simulink model "LV"  (R2016a)
settings: Solver=VariableStepAuto  StartTime=0.0  StopTime=10.0  RelTol=1e-3
libraries: powerlib x22
settings Model: Creator=Hp  LastModifiedBy=Hp

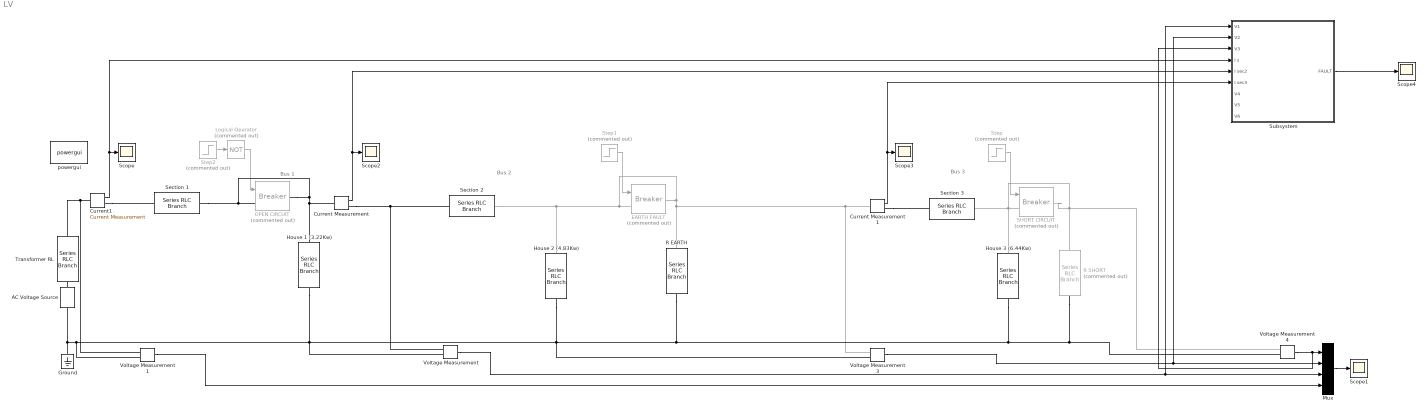
== system LV ==
  note: Bus 3
  note: Bus 2
  note: Bus 1
  AC Voltage Source : powerlib/Electrical Sources/AC Voltage Source  Amplitude=230  Phase=0  Frequency=50  SampleTime=0  Measurements=Voltage  BusType=swing  Pref=10e3  Qref=0  Qmin=-inf  Qmax=+inf
  Current Measurement : powerlib/Measurements/Current Measurement  PhasorSimulation=off  OutputType=Complex  PSBequivalent=0
  Current Measurement1 : powerlib/Measurements/Current Measurement  PhasorSimulation=off  OutputType=Complex  PSBequivalent=0
  Current1 : powerlib/Measurements/Current Measurement  PhasorSimulation=off  OutputType=Complex  PSBequivalent=0
  EARTH FAULT : powerlib/Elements/Breaker  Commented=on  InitialState=0  SwitchingTimes="[1/60  5/60]"  External=on  BreakerResistance=0.05  SnubberResistance=1e6  SnubberCapacitance=inf  Measurements=None  MoreParameters=on  NoBreakLoop=off
  Ground : powerlib/Elements/Ground  LConnTagsString=a
  House 1 (3.22Kw) : powerlib/Elements/Series RLC Branch  LConnTagsString=__new0  RConnTagsString=__new0  BranchType=RL  Resistance=16.43  Inductance=0.02497  SetiL0=off  InitialCurrent=0  Capacitance=1e-6  Setx0=off  InitialVoltage=0  Measurements=None
  House 2 (4.83Kw) : powerlib/Elements/Series RLC Branch  LConnTagsString=__new0  RConnTagsString=__new0  BranchType=RL  Resistance=10.95  Inductance=0.01665  SetiL0=off  InitialCurrent=0  Capacitance=1e-6  Setx0=off  InitialVoltage=0  Measurements=None
  House 3 (6.44Kw) : powerlib/Elements/Series RLC Branch  LConnTagsString=__new0  RConnTagsString=__new0  BranchType=RL  Resistance=8.21  Inductance=0.01249  SetiL0=off  InitialCurrent=0  Capacitance=1e-6  Setx0=off  InitialVoltage=0  Measurements=None
  Logical Operator : Logic  Commented=on  Operator=NOT  AllPortsSameDT=off  OutDataTypeStr=boolean
  Mux : Mux
  OPEN CIRCUIT : powerlib/Elements/Breaker  Commented=on  InitialState=0  SwitchingTimes="[1/60  5/60]"  External=on  BreakerResistance=0.05  SnubberResistance=1e6  SnubberCapacitance=inf  Measurements=None  MoreParameters=on  NoBreakLoop=off
  R EARTH : powerlib/Elements/Series RLC Branch  LConnTagsString=__new0  RConnTagsString=__new0  BranchType=R  Resistance=0.1  Inductance=0.01249  SetiL0=off  InitialCurrent=0  Capacitance=1e-6  Setx0=off  InitialVoltage=0  Measurements=None
  R SHORT : powerlib/Elements/Series RLC Branch  Commented=on  LConnTagsString=__new0  RConnTagsString=__new0  BranchType=R  Resistance=0.01  Inductance=0.01249  SetiL0=off  InitialCurrent=0  Capacitance=1e-6  Setx0=off  InitialVoltage=0  Measurements=None
  SHORT CIRCUIT : powerlib/Elements/Breaker  Commented=on  InitialState=0  SwitchingTimes="[1/60  5/60]"  External=on  BreakerResistance=0.01  SnubberResistance=1e6  SnubberCapacitance=inf  Measurements=None  MoreParameters=on  NoBreakLoop=off
  Scope{,1..4} (5 alike) : Scope
  Section 1 : powerlib/Elements/Series RLC Branch  LConnTagsString=__new0  RConnTagsString=__new0  BranchType=RL  Resistance=0.05  Inductance=0.001  SetiL0=off  InitialCurrent=0  Capacitance=1e-6  Setx0=off  InitialVoltage=0  Measurements=None
  Section 2 : powerlib/Elements/Series RLC Branch  LConnTagsString=__new0  RConnTagsString=__new0  BranchType=RL  Resistance=0.05  Inductance=0.001  SetiL0=off  InitialCurrent=0  Capacitance=1e-6  Setx0=off  InitialVoltage=0  Measurements=None
  Section 3 : powerlib/Elements/Series RLC Branch  LConnTagsString=__new0  RConnTagsString=__new0  BranchType=RL  Resistance=0.05  Inductance=0.001  SetiL0=off  InitialCurrent=0  Capacitance=1e-6  Setx0=off  InitialVoltage=0  Measurements=None
  Step : Step  Commented=on  Time=0  SampleTime=0
  Step1 : Step  Commented=on  Time=0  SampleTime=0
  Step2 : Step  Commented=on  Time=0  SampleTime=0
  Subsystem : Subsystem
  "Transformer RL " : powerlib/Elements/Series RLC Branch  LConnTagsString=__new0  RConnTagsString=__new0  BranchType=RL  Resistance=0.0001  Inductance=0.000000001  SetiL0=off  InitialCurrent=0  Capacitance=1e-6  Setx0=off  InitialVoltage=0  Measurements=None
  Voltage Measurement{,1,3..4} (4 alike) : powerlib/Measurements/Voltage Measurement  PhasorSimulation=off  OutputType=Complex  PSBequivalent=0
  powergui : powerlib/powergui  Priority=1  SimulationMode=Discrete  SolverType=Tustin/Backward Euler (TBE)  SampleTime=5e-5  frequency=60  SPID=off  DisableSnubberDevices=off  DisableRonSwitches=off  DisableVfSwitches=off  SwTol=0  DisplayEquations=off  Interpol=off  ExternalGateDelay=off  methode=off  Ts=10  FunctionMessages=off  echomessages=off  HookPort=off  EnableUseOfTLC=off  x0status=blocks  frequencyindice=50  Pbase=100e6  ErrMax=1e-4  Iterations=50  UnitsV=kV  UnitsW=MW  buscounter=0  RestoreLinks=warning  ResistiveCurrentMeasurement=off  Frange=[0:2:500]  Ylog=off  Xlog=on  ShowGrid=off  save=off  variable=ZData  structure=0  ZoomFFT=off  StartTime=0.0  cycles=1  DisplayStyle=1  fundamental=60  FreqAxis=off  MaxFrequency=1000  frequencyindicesteady=1  RmsSteady=1  display=off
  wires:
  Voltage Measurement4/1 -> Subsystem/3(V3), Mux/1
  Mux/1 -> Scope1/1
  Voltage Measurement1/1 -> Mux/4
  Voltage Measurement/1 -> Subsystem/1(V1), Mux/3
  Voltage Measurement3/1 -> Subsystem/2(V2), Mux/2
  Current Measurement/1 -> Subsystem/5(I sec2), Scope2/1
  Current Measurement1/1 -> Subsystem/6(I sec3), Scope3/1
  Current1/1 -> Subsystem/4(I s), Scope/1
  Step/1 -> SHORT CIRCUIT/1
  Step1/1 -> EARTH FAULT/1
  Step2/1 -> Logical Operator/1
  Logical Operator/1 -> OPEN CIRCUIT/1
  Subsystem/1(FAULT) -> Scope4/1
  connections:
  EARTH FAULT/RConn1 -- Voltage Measurement3/LConn1 -- Current Measurement1/LConn1 -- R EARTH/LConn1 -- Section 2/RConn1 -- House 2 (4.83Kw)/LConn1 -- EARTH FAULT/LConn1
  Voltage Measurement1/LConn1 -- Current1/LConn1 -- "Transformer RL "/RConn1
  Current Measurement/RConn1 -- Voltage Measurement/LConn1 -- Section 2/LConn1
  SHORT CIRCUIT/RConn1 -- Voltage Measurement4/LConn1 -- House 3 (6.44Kw)/LConn1 -- SHORT CIRCUIT/LConn1 -- Section 3/RConn1 -- R SHORT/LConn1
  Current1/RConn1 -- Section 1/LConn1
  "Transformer RL "/LConn1 -- AC Voltage Source/RConn1
  Current Measurement1/RConn1 -- Section 3/LConn1
  House 3 (6.44Kw)/RConn1 -- House 1 (3.22Kw)/RConn1 -- AC Voltage Source/LConn1 -- Ground/LConn1 -- Voltage Measurement1/LConn2 -- Voltage Measurement/LConn2 -- House 2 (4.83Kw)/RConn1 -- Voltage Measurement3/LConn2 -- R EARTH/RConn1 -- Voltage Measurement4/LConn2 -- R SHORT/RConn1
  House 1 (3.22Kw)/LConn1 -- OPEN CIRCUIT/RConn1 -- Section 1/RConn1 -- OPEN CIRCUIT/LConn1 -- Current Measurement/LConn1

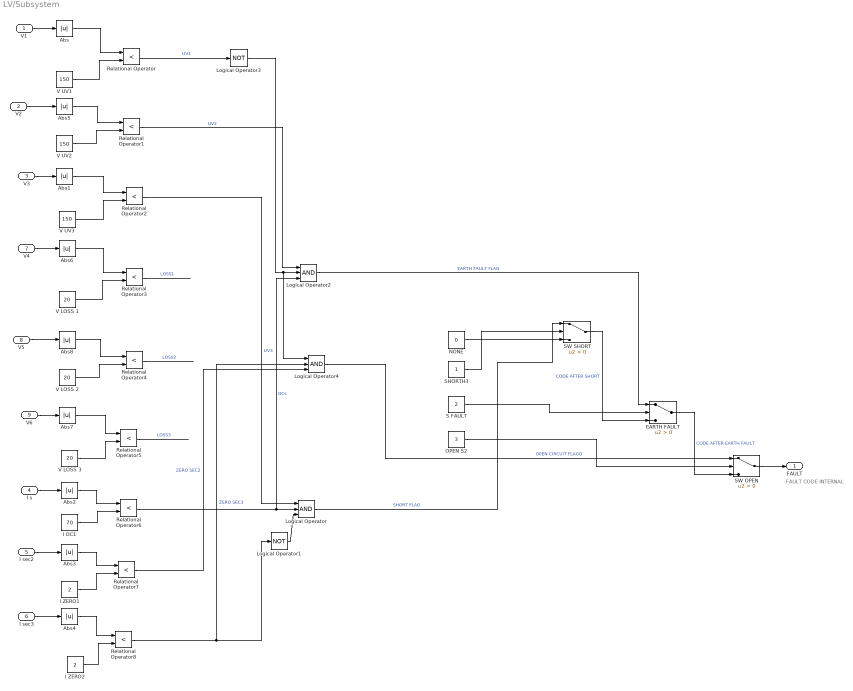
== system LV/Subsystem ==
  note: FAULT CODE INTERNAL
  V1 : Inport
  V2 : Inport  Port=2
  V3 : Inport  Port=3
  I s : Inport  Port=4
  I sec2 : Inport  Port=5
  I sec3 : Inport  Port=6
  V4 : Inport  Port=7
  V5 : Inport  Port=8
  V6 : Inport  Port=9
  Abs{,1..8} (9 alike) : Abs
  EARTH FAULT : Switch  Criteria=u2 > Threshold
  I OC1 : Constant  Value=70
  I ZERO1 : Constant  Value=2
  I ZERO2 : Constant  Value=2
  Logical Operator : Logic  Inputs=3  AllPortsSameDT=off  OutDataTypeStr=boolean
  Logical Operator1 : Logic  Operator=NOT  Inputs=3  AllPortsSameDT=off  OutDataTypeStr=boolean
  Logical Operator2 : Logic  Inputs=3  AllPortsSameDT=off  OutDataTypeStr=boolean
  Logical Operator3 : Logic  Operator=NOT  Inputs=3  AllPortsSameDT=off  OutDataTypeStr=boolean
  Logical Operator4 : Logic  Inputs=3  AllPortsSameDT=off  OutDataTypeStr=boolean
  NONE : Constant  Value=0
  OPEN S2 : Constant  Value=3
  Relational Operator{,1..8} (9 alike) : RelationalOperator  Operator=<  OutDataTypeStr=boolean
  S FAULT : Constant  Value=2
  SHORTH3 : Constant
  SW OPEN : Switch  Criteria=u2 > Threshold
  SW SHORT : Switch  Criteria=u2 > Threshold
  V LOSS 1 : Constant  Value=20
  V LOSS 2 : Constant  Value=20
  V LOSS 3 : Constant  Value=20
  V UV1 : Constant  Value=150
  V UV2 : Constant  Value=150
  V UV3 : Constant  Value=150
  FAULT : Outport
  wires:
  V2/1 -> Abs5/1
  V3/1 -> Abs1/1
  I s/1 -> Abs2/1
  I sec2/1 -> Abs3/1
  I sec3/1 -> Abs4/1
  Abs5/1 -> Relational Operator1/1
  Abs1/1 -> Relational Operator2/1
  Abs2/1 -> Relational Operator6/1
  Abs3/1 -> Relational Operator7/1
  Abs4/1 -> Relational Operator8/1
  V1/1 -> Abs/1
  Abs/1 -> Relational Operator/1
  V UV1/1 -> Relational Operator/2
  Relational Operator/1 -> Logical Operator3/1  "UV1"
  V UV2/1 -> Relational Operator1/2
  V UV3/1 -> Relational Operator2/2
  V5/1 -> Abs8/1
  V6/1 -> Abs7/1
  Abs8/1 -> Relational Operator4/1
  Abs7/1 -> Relational Operator5/1
  V4/1 -> Abs6/1
  Abs6/1 -> Relational Operator3/1
  V LOSS 1/1 -> Relational Operator3/2
  Relational Operator3/1 -> ?  "LOSS1"
  V LOSS 2/1 -> Relational Operator4/2
  V LOSS 3/1 -> Relational Operator5/2
  I OC1/1 -> Relational Operator6/2
  I ZERO1/1 -> Relational Operator7/2
  I ZERO2/1 -> Relational Operator8/2
  Relational Operator4/1 -> ?  "LOSS2"
  Relational Operator5/1 -> ?  "LOSS3"
  Relational Operator1/1 -> Logical Operator2/1  "UV2"
  Relational Operator2/1 -> Logical Operator/1  "UV3"
  Relational Operator6/1 -> Logical Operator2/3, Logical Operator/2  "OCs"
  Relational Operator7/1 -> Logical Operator4/3  "ZERO SEC2"
  Relational Operator8/1 -> Logical Operator4/2, Logical Operator1/1  "ZERO SEC3"
  Logical Operator1/1 -> Logical Operator/3
  Logical Operator/1 -> SW SHORT/1  "SHORT FLAG"
  Logical Operator3/1 -> Logical Operator4/1, Logical Operator2/2
  Logical Operator2/1 -> EARTH FAULT/1  "EARTH FAULT FLAG"
  Logical Operator4/1 -> SW OPEN/1  "OPEN CIRCUIT FLAGG"
  SHORTH3/1 -> SW SHORT/2
  NONE/1 -> SW SHORT/3
  SW SHORT/1 -> EARTH FAULT/3  "CODE AFTER SHORT"
  S FAULT/1 -> EARTH FAULT/2
  OPEN S2/1 -> SW OPEN/2
  EARTH FAULT/1 -> SW OPEN/3  "CODE AFTER EARTH FAULT"
  SW OPEN/1 -> FAULT/1
